simulink model "Sim_PMSMCtrl"  (R2023a)
settings: Solver=FixedStepDiscrete  StartTime=0.0  StopTime=0.3  RelTol=1e-3
PreLoadFcn:
  | addpath("Sim\")
  | Sim_PreLoad_PMSMCtrl;
undefined symbols (not defined in the file): Hw_Par_fTpwm, Hw_Par_fVdc, Mt_Par_fF, Mt_Par_fInitTheta, Mt_Par_fJ, Mt_Par_fLd, Mt_Par_fLq, Mt_Par_fNp, Mt_Par_fRs, Mt_Par_fTf, Sim_Par_fSysTs
libraries: Lib_General x2, simulink x2, spsDCVoltageSourceLib x1, spsPermanentMagnetSynchronousMachineLib x1, spsUniversalBridgeLib x1, spsVoltageMeasurementLib x1, sps_lib x1
settings Model: Creator=62555  LastModifiedBy=62555
settings OptimizationCC: DefaultParameterBehavior=Inlined  UseDivisionForNetSlopeComputation=on  DefaultUnderspecifiedDataType=single  EnhancedBackFolding=on  PassReuseOutputArgsAs=Individual arguments  ZeroExternalMemoryAtStartup=off  ZeroInternalMemoryAtStartup=off  OptimizeBlockOrder=speed  DifferentSizesBufferReuse=on  OptimizationCustomize=off  EfficientTunableParamExpr=on
settings DebuggingCC: ParameterTunabilityLossMsg=error
settings SFSimCC: MATLABDynamicMemAlloc=off
settings RTWCC: Description=Embedded Coder  SystemTargetFile=ert.tlc  GenCodeOnly=on  TemplateMakefile=ert_default_tmf  GenerateReport=on  LaunchReport=on
settings CodeAppCC: ForceParamTrailComments=on  IgnoreCustomStorageClasses=off  OperatorAnnotations=on  SimulinkDataObjDesc=on  SFDataObjDesc=on  InsertBlockDesc=on
settings ERTTargetCC: TargetLangStandard=C99 (ISO)  GenerateSampleERTMain=on  InlinedParameterPlacement=NonHierarchical  ERTCustomFileTemplate=example_file_process.tlc

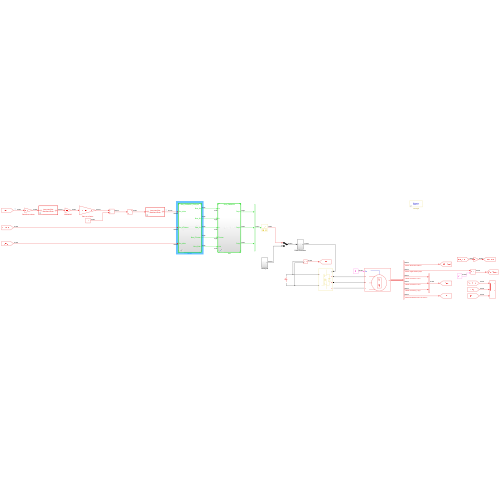
[thumbnail: Simulink's stored preview of the top-level diagram]
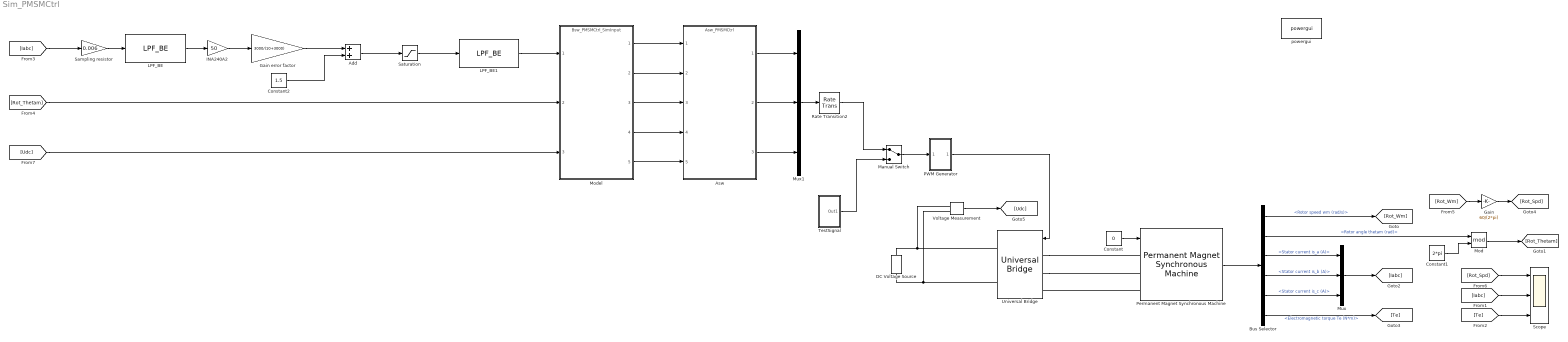
== system Sim_PMSMCtrl ==
  Add : Sum
  Asw : ModelReference  ModelNameDialog=Asw_PMSMCtrl.slx  SimulationMode=Normal  ModelReferenceVersion=1.170
  Bus Selector : BusSelector  OutputSignals=Rotor speed wm (rad/s),Rotor angle thetam (rad),Stator current is_a (A),Stator current is_b (A),Stator current is_c (A),Electromagnetic torque Te (N*m)
  Constant : Constant  Value=0  OutDataTypeStr=double
  Constant1 : Constant  Value=2*pi  OutDataTypeStr=double
  Constant2 : Constant  Value=1.5  SampleTime=-1
  DC Voltage Source : spsDCVoltageSourceLib/DC Voltage Source  Amplitude=double(Hw_Par_fVdc)  Measurements=None
  Gain : Gain  Gain=60/(2*pi)
  Gain error factor : Gain  Gain=3000/(10+3000)
  INA240A2 : Gain  Gain=50
  LPF_BE : Lib_General/LPF_BE  tau=2*10*1.5e-9  Ts=Sim_Par_fSysTs  Initial_condition=0
      settings: SourceProductName=Lib_PE
  LPF_BE1 : Lib_General/LPF_BE  tau=1e3*1e-9  Ts=Sim_Par_fSysTs  Initial_condition=0
      settings: SourceProductName=Lib_PE
  Manual Switch : ManualSwitch
  Mod : Math  Operator=mod
  Model : ModelReference  ModelNameDialog=Bsw_PMSMCtrl_SimInput.slx  SimulationMode=Normal  ModelReferenceVersion=1.85
  Mux : Mux  Inputs=3
  Mux1 : Mux  Inputs=3
  PWM Generator : Subsystem
  Permanent Magnet Synchronous Machine : spsPermanentMagnetSynchronousMachineLib/Permanent Magnet Synchronous Machine  NbPhases=3  FluxDistribution=Sinusoidal  RotorType=Salient-pole  MechanicalLoad=Torque Tm  PresetModel=No  ShowDetailedParameters=on  MeasurementBus=off  Resistance=Mt_Par_fRs  Inductance=8.5e-3  dqInductances=[Mt_Par_fLd,Mt_Par_fLq]  La=0.000395  MachineConstant=Flux linkage established by magnets (V.s)  Flux=Mt_Par_fFlux  VoltageCst=13.3012  TorqueCst=0.11  Flat=120  Mechanical=[Mt_Par_fJ Mt_Par_fF Mt_Par_fNp Mt_Par_fTf]  PolePairs=4  InitialConditions=[0,Mt_Par_fInitTheta, 0,0]  InitialConditions5ph=[0 0 0 0 0 0]  RefAngle=Aligned with phase A axis (original Park)  IterativeDiscreteModel=Trapezoidal non iterative  TsBlock=-1  TsPowergui=0
  Rate Transition2 : RateTransition
  Sampling resistor : Gain  Gain=0.006
  Saturation : Saturate  UpperLimit=3  LowerLimit=0
  Scope : Scope  NumInputPorts=3
  TestSignal : Subsystem
  Universal Bridge : spsUniversalBridgeLib/Universal Bridge  Arms=3  SnubberResistance=1e5  SnubberCapacitance=inf  Device=MOSFET / Diodes  Ron=Hw_Par_fRon  Lon=0  ForwardVoltages="[  0  0  ]"  ForwardVoltage=0  GTOparameters=[ 10e-6 , 20e-6 ]  IGBTparameters=[ 1e-6 , 2e-6 ]  Measurements=None  Measurements_2=None  converterType=Rectifier
  Voltage Measurement : spsVoltageMeasurementLib/Voltage Measurement  PhasorSimulation=off  OutputType=Complex  PSBequivalent=0
  powergui : sps_lib/powergui  Priority=1  SimulationMode=Discrete  SampleTime=Sim_Par_fSysTs  frequency=60  Iterations=50  frequencyindice=0  Pbase=100e6  ErrMax=1e-4  UnitsV=kV  UnitsW=MW  buscounter=0  FunctionMessages=off  echomessages=off  EnableUseOfTLC=off  CurrentSourceSwitches=off  DisableSnubberDevices=off  DisableRonSwitches=off  DisableVfSwitches=off  DisplayEquations=off  AutomaticDiscreteSolvers=off  SolverType=Tustin/Backward Euler (TBE)  Interpol=off  ExternalGateDelay=off  methode=off  Ts=100  x0status=blocks  SPID=on  SwTol=0  HookPort=off  NonlinearTolerance=1e-4  nMaxIteration=100  ContinueOnMaxIteration=off  RestoreLinks=warning  ResistiveCurrentMeasurement=off  Frange=[0:2:500]  Ylog=off  Xlog=on  ShowGrid=off  save=off  variable=ZData  structure=0  ZoomFFT=off  StartTime=0.0  cycles=1  DisplayStyle=1  fundamental=60  FreqAxis=off  MaxFrequency=1000  frequencyindicesteady=1  RmsSteady=1  display=off
  wires:
  Permanent Magnet Synchronous Machine/1 -> Bus Selector/1
  Bus Selector/1 -> [Rot_Wm]  "<Rotor speed wm (rad/s)>"
  Bus Selector/2 -> Mod/1  "<Rotor angle thetam (rad)>"
  Bus Selector/3 -> Mux/1  "<Stator current is_a (A)>"
  Bus Selector/4 -> Mux/2  "<Stator current is_b (A)>"
  Bus Selector/5 -> Mux/3  "<Stator current is_c (A)>"
  Bus Selector/6 -> [Te]  "<Electromagnetic torque Te (N*m)>"
  Mux/1 -> [Iabc]
  Constant/1 -> Permanent Magnet Synchronous Machine/1
  [Rot_Spd] -> Scope/1
  [Iabc] -> Scope/2
  [Te] -> Scope/3
  TestSignal/1(Out1) -> Manual Switch/2
  PWM Generator/1(Out1) -> Universal Bridge/1
  Manual Switch/1 -> PWM Generator/1(In1)
  Constant1/1 -> Mod/2
  Mod/1 -> [Rot_Thetam]
  [Rot_Thetam] -> Model/2
  Asw/1 -> Mux1/1
  Asw/2 -> Mux1/2
  Asw/3 -> Mux1/3
  Mux1/1 -> Rate Transition2/1
  [Rot_Wm] -> Gain/1
  Gain/1 -> [Rot_Spd]
  Rate Transition2/1 -> Manual Switch/1
  Voltage Measurement/1 -> [Udc]
  [Udc] -> Model/3
  Model/5 -> Asw/5
  Model/4 -> Asw/4
  Model/3 -> Asw/3
  Model/2 -> Asw/2
  Model/1 -> Asw/1
  INA240A2/1 -> Gain error factor/1
  LPF_BE/1 -> INA240A2/1
  Sampling resistor/1 -> LPF_BE/1
  [Iabc] -> Sampling resistor/1
  Gain error factor/1 -> Add/1
  LPF_BE1/1 -> Model/1
  Add/1 -> Saturation/1
  Constant2/1 -> Add/2
  Saturation/1 -> LPF_BE1/1
  connections:
  Universal Bridge/LConn1 -- Permanent Magnet Synchronous Machine/LConn1
  Universal Bridge/LConn2 -- Permanent Magnet Synchronous Machine/LConn2
  Permanent Magnet Synchronous Machine/LConn3 -- Universal Bridge/LConn3
  DC Voltage Source/RConn1 -- Voltage Measurement/LConn1 -- Universal Bridge/RConn1
  Universal Bridge/RConn2 -- Voltage Measurement/LConn2 -- DC Voltage Source/LConn1

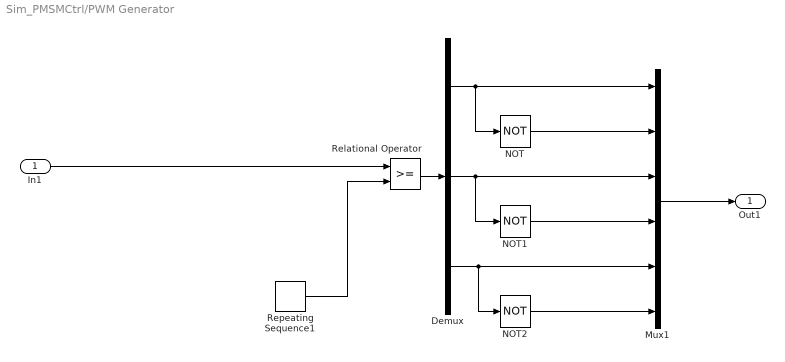
== system Sim_PMSMCtrl/PWM Generator ==
  In1 : Inport
  Demux : Demux  Outputs=3
  Mux1 : Mux  Inputs=6
  NOT : Logic  Operator=NOT  IconShape=distinctive  AllPortsSameDT=off  OutDataTypeStr=boolean
  NOT1 : Logic  Operator=NOT  IconShape=distinctive  AllPortsSameDT=off  OutDataTypeStr=boolean
  NOT2 : Logic  Operator=NOT  IconShape=distinctive  AllPortsSameDT=off  OutDataTypeStr=boolean
  Relational Operator : RelationalOperator  OutDataTypeStr=boolean  RndMeth=Simplest  InputSameDT=off
  Repeating Sequence1 : simulink/Sources/Repeating Sequence  rep_seq_t=[0 Hw_Par_fTpwm/2 Hw_Par_fTpwm]  rep_seq_y=[0 1 0]
  Out1 : Outport
  wires:
  Demux/1 -> Mux1/1, NOT/1
  Demux/3 -> NOT2/1, Mux1/5
  Demux/2 -> NOT1/1, Mux1/3
  NOT2/1 -> Mux1/6
  NOT/1 -> Mux1/2
  Repeating Sequence1/1 -> Relational Operator/2
  NOT1/1 -> Mux1/4
  Relational Operator/1 -> Demux/1
  Mux1/1 -> Out1/1
  In1/1 -> Relational Operator/1

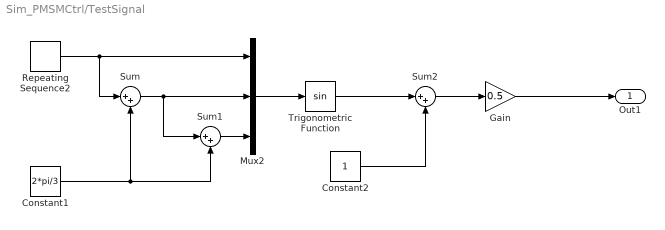
== system Sim_PMSMCtrl/TestSignal ==
  Constant1 : Constant  Value=2*pi/3  OutDataTypeStr=double
  Constant2 : Constant  OutDataTypeStr=double
  Gain : Gain  Gain=0.5
  Mux2 : Mux  Inputs=3
  Repeating Sequence2 : simulink/Sources/Repeating Sequence  rep_seq_t=[0 Hw_Par_fTpwm*100]  rep_seq_y=[0 2*pi]
  Sum : Sum  Inputs=|++
  Sum1 : Sum  Inputs=|++
  Sum2 : Sum  Inputs=|++
  Trigonometric Function : Trigonometry
  Out1 : Outport
  wires:
  Sum/1 -> Sum1/1, Mux2/2
  Constant1/1 -> Sum1/2, Sum/2
  Sum2/1 -> Gain/1
  Sum1/1 -> Mux2/3
  Constant2/1 -> Sum2/2
  Mux2/1 -> Trigonometric Function/1
  Trigonometric Function/1 -> Sum2/1
  Repeating Sequence2/1 -> Mux2/1, Sum/1
  Gain/1 -> Out1/1
